simulink model "gm_sampleModel1580_4_sub"  (R2023a)
settings: Solver=VariableStepAuto  StartTime=0.0  StopTime=10.0  RelTol=1e-3
libraries: hdlsllib x3, simulink x2
settings Model: Creator=user1  LastModifiedBy=user1
settings OptimizationCC: BlockReduction=off  ConditionallyExecuteInputs=off
settings DebuggingCC: InheritedTsInSrcMsg=none

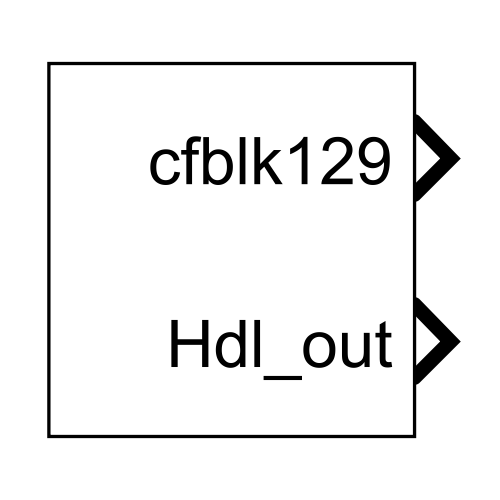
[thumbnail: Simulink's stored preview of the top-level diagram]
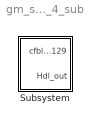
== system gm_sampleModel1580_4_sub ==
  Subsystem : Subsystem

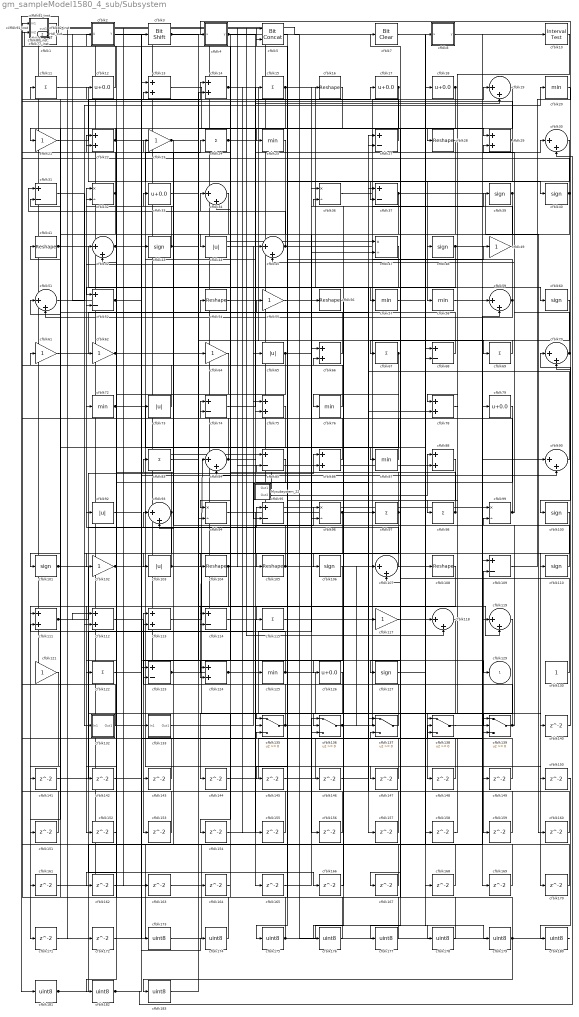
== system gm_sampleModel1580_4_sub/Subsystem ==
  Mysubsystem_22 : Subsystem
  cfblk1 : simulink/Logic and Bit Operations/Bit Clear  iBit=0
      settings: LibrarySourceBlock=|
      | hdlsllib/Logic and Bit
      | Operations/Bit Clear
  cfblk10 : hdlsllib/Logic and Bit Operations/Interval Test  IntervalClosedRight=on  uplimit=0.5  IntervalClosedLeft=on  lowlimit=-0.5  OutDataTypeStr=uint8
  cfblk{39..40,43,48,60,100..101,106,110,127} (10 alike) : Signum
  cfblk{21,23,49,55,61..62,64,102,117,121} (10 alike) : Gain  OutDataTypeStr=uint8
  cfblk{44,65,73,92,103} (5 alike) : Abs  OutDataTypeStr=uint8  SaturateOnIntegerOverflow=off
  cfblk{16,28,41,54,56,104..105,108} (8 alike) : Reshape
  cfblk{19,30,34,42,45,51,59,70,84,90,93,107,118..119} (14 alike) : Sum  Inputs=|++  OutDataTypeStr=uint8
  cfblk{27,31,37,52,68,74,85,95,109,114,123} (11 alike) : Sum  Inputs=+-  OutDataTypeStr=uint8
  cfblk{11,15,24,67,69,83,97..98,115,122} (10 alike) : Sum  Inputs=+  OutDataTypeStr=uint8
  cfblk{13..14,22,29,66,75,78,86,88,111..113,124} (13 alike) : Sum  OutDataTypeStr=uint8
  cfblk{12,17..18,33,79,126} (6 alike) : Bias  Bias=0.0  SaturateOnIntegerOverflow=off
  cfblk120_inst : Subsystem
  cfblk{20,25,57..58,72,76,87,125} (8 alike) : MinMax  OutDataTypeStr=uint8
  cfblk130 : Constant  OutDataTypeStr=uint8  SampleTime=-1
  cfblk132 : Subsystem
  cfblk133 : Subsystem
  cfblk{135..139} (5 alike) : Switch  OutDataTypeStr=uint8  SaturateOnIntegerOverflow=off  InputSameDT=off
  cfblk{140..172} (33 alike) : Delay  SampleTime=1
  cfblk{173..183} (11 alike) : DataTypeConversion  OutDataTypeStr=uint8  SaturateOnIntegerOverflow=off  RndMeth=Floor
  cfblk2 : Subsystem  mask(Detect Rise Nonnegative){vinit=double(0), InputProcessing=Elements as channels (sample based), OutDataTypeStr=uint8}
      mask prompts: vinit "Simulink:masks:InitialCondition_MP"; InputProcessing "Simulink:masks:InputProcessing_MP"; OutDataTypeStr "Simulink:masks:OutputDataType_MP"
      mask help: Simulink:masks:DetectRiseNonnegative_MD
      mask init:
      | InputProcessing = 'Elements as channels (sample based)';
      | OutDataTypeStr = 'uint8';
      | vinit = double(0);
      mask TypeOptions InputProcessing: Simulink:masks:ColumnsAsChannelsFrameBased | Simulink:masks:ElementsAsChannelsSampleBased
      mask TypeOptions OutDataTypeStr: Simulink:masks:uint8 | Simulink:masks:boolean
      mask Display: fprintf('U >= 0\n&  NOT\nU/z >= 0')
  cfblk3 : hdlsllib/Logic and Bit Operations/Bit Shift  mode=Shift Left Logical  N=0
  cfblk{32,36,47,94,96,99} (6 alike) : Product  Inputs=*/  OutDataTypeStr=uint8  RndMeth=Zero  SaturateOnIntegerOverflow=on
  cfblk4 : Subsystem  mask(Compare To Zero){relop=<=, OutDataTypeStr=uint8, ZeroCross=on}
      mask prompts: relop "Simulink:masks:Operator_MP"; OutDataTypeStr "Simulink:masks:OutputDataType_MP"; ZeroCross "Simulink:masks:EnableZerocrossingDetection_MP"
      mask help: Simulink:masks:CompareToZero_MD
      mask init:
      | OutDataTypeStr = 'uint8';
      | ZeroCross = 'on';
      | blkName = 'sampleModel1580_4_sub/Subsystem/cfblk4';
      | relop = '<=';
      | setValue = 'fixdt(0, 8)';
      mask TypeOptions relop: == | ~= | < | <= | >= | >
      mask TypeOptions OutDataTypeStr: Simulink:masks:uint8 | Simulink:masks:boolean
      mask Callback ZeroCross: sl('zeroCrossEnable', gcbh);
      mask Display: disp([relop,' 0'])
  cfblk46_inst : Subsystem
  cfblk5 : hdlsllib/Logic and Bit Operations/Bit Concat  numInputs=2
  cfblk50_inst : Subsystem
  cfblk53_inst : Subsystem
  cfblk6 : Constant  Value=0  OutDataTypeStr=uint8  SampleTime=1
  cfblk63_inst : Subsystem
  cfblk7 : simulink/Logic and Bit Operations/Bit Clear  iBit=0
      settings: LibrarySourceBlock=|
      | hdlsllib/Logic and Bit
      | Operations/Bit Clear
  cfblk71_inst : Subsystem
  cfblk77_inst : Subsystem
  cfblk8 : Subsystem  mask(Compare To Constant){relop=<=, const=double(3), OutDataTypeStr=uint8, ZeroCross=on}
      mask prompts: relop "Simulink:masks:Operator_MP"; const "Simulink:masks:ConstantValue_MP"; OutDataTypeStr "Simulink:masks:OutputDataType_MP"; ZeroCross "Simulink:masks:EnableZerocrossingDetection_MP"
      mask help: Simulink:masks:CompareToConstant_MD
      mask init:
      | OutDataTypeStr = 'uint8';
      | ZeroCross = 'on';
      | blkName = 'sampleModel1580_4_sub/Subsystem/cfblk8';
      | const = double(3);
      | const_str = '3.0';
      | const_val = double(3);
      | relop = '<=';
      | setValue = 'fixdt(0, 8)';
      | str = '<= 3';
      mask TypeOptions relop: == | ~= | < | <= | >= | >
      mask TypeOptions OutDataTypeStr: Simulink:masks:uint8 | Simulink:masks:boolean
      mask Callback ZeroCross: sl('zeroCrossEnable', gcbh);
      mask Display: disp(str)
  cfblk80_inst : Subsystem
  cfblk81_inst : Subsystem
  cfblk82_inst : Subsystem
  cfblk9 : Constant  Value=0  OutDataTypeStr=uint8  SampleTime=1
  cfblk91_inst : Subsystem
  cfblk129 : Outport  OutDataTypeStr=uint8  SampleTime=1  VectorParamsAs1DForOutWhenUnconnected=off
  Hdl_out : Outport  Port=2  OutDataTypeStr=uint8  SampleTime=1
  wires:
  Mysubsystem_22/1(Out1) -> cfblk80_inst/2(in2)
  Mysubsystem_22/2(Out2) -> cfblk88/1
  cfblk1/1 -> cfblk181/1
  cfblk10/1 -> cfblk135/1
  cfblk100/1 -> cfblk170/1
  cfblk101/1 -> cfblk86/1, cfblk136/2, cfblk166/1
  cfblk102/1 -> cfblk150/1, cfblk24/1
  cfblk103/1 -> cfblk32/1, cfblk140/1
  cfblk104/1 -> cfblk75/1, cfblk152/1
  cfblk105/1 -> cfblk33/1, cfblk61/1
  cfblk106/1 -> cfblk153/1
  cfblk107/1 -> cfblk92/1
  cfblk108/1 -> cfblk171/1
  cfblk109/1 -> cfblk4/1(u)
  cfblk11/1 -> cfblk58/1
  cfblk110/1 -> cfblk83/1
  cfblk111/1 -> cfblk95/1, cfblk112/1
  cfblk112/1 -> cfblk143/1
  cfblk113/1 -> cfblk115/1
  cfblk114/1 -> cfblk165/1
  cfblk115/1 -> cfblk49/1
  cfblk117/1 -> cfblk18/1
  cfblk118/1 -> cfblk148/1
  cfblk119/1 -> cfblk144/1
  cfblk12/1 -> cfblk82_inst/1(in1)
  cfblk120_inst/1(out1) -> cfblk91_inst/1(in1), cfblk118/2, cfblk133/1(In1)
  cfblk121/1 -> cfblk161/1
  cfblk122/1 -> cfblk3/1
  cfblk123/1 -> cfblk84/1, cfblk136/3
  cfblk124/1 -> cfblk56/1, cfblk159/1
  cfblk125/1 -> cfblk111/2, cfblk168/1
  cfblk126/1 -> cfblk154/1
  cfblk127/1 -> cfblk8/1(u)
  cfblk13/1 -> cfblk75/2
  cfblk130/1 -> cfblk85/2
  cfblk132/1(Out1) -> cfblk50_inst/1(in1)
  cfblk133/1(Out1) -> cfblk65/1
  cfblk135/1 -> cfblk54/1, cfblk147/1
  cfblk136/1 -> cfblk19/1, cfblk107/1
  cfblk137/1 -> cfblk113/1
  cfblk138/1 -> cfblk109/2
  cfblk139/1 -> cfblk123/2, cfblk99/2
  cfblk14/1 -> cfblk156/1, cfblk155/1
  cfblk140/1 -> cfblk70/1
  cfblk141/1 -> cfblk45/1
  cfblk142/1 -> cfblk90/2
  cfblk143/1 -> cfblk51/1
  cfblk144/1 -> cfblk137/3
  cfblk145/1 -> cfblk109/1
  cfblk146/1 -> cfblk27/2
  cfblk147/1 -> cfblk93/1
  cfblk148/1 -> cfblk107/2
  cfblk149/1 -> cfblk46_inst/1(in1)
  cfblk15/1 -> cfblk52/1, cfblk157/1
  cfblk150/1 -> cfblk180/1
  cfblk151/1 -> cfblk53_inst/2(in2)
  cfblk152/1 -> cfblk32/2
  cfblk153/1 -> cfblk77_inst/1(in1)
  cfblk154/1 -> cfblk96/1
  cfblk155/1 -> cfblk74/1
  cfblk156/1 -> cfblk120_inst/1(in1)
  cfblk157/1 -> cfblk137/1
  cfblk158/1 -> cfblk138/2
  cfblk159/1 -> cfblk138/3
  cfblk16/1 -> cfblk25/1
  cfblk160/1 -> cfblk36/2
  cfblk161/1 -> cfblk123/1
  cfblk162/1 -> cfblk68/1
  cfblk163/1 -> cfblk59/2
  cfblk164/1 -> cfblk84/2
  cfblk165/1 -> cfblk136/1
  cfblk166/1 -> cfblk66/2
  cfblk167/1 -> cfblk50_inst/2(in2)
  cfblk168/1 -> cfblk81_inst/2(in2)
  cfblk169/1 -> cfblk31/2
  cfblk17/1 -> cfblk34/2, cfblk101/1
  cfblk170/1 -> cfblk113/2
  cfblk171/1 -> cfblk139/2
  cfblk172/1 -> cfblk139/1
  cfblk173/1 -> cfblk79/1
  cfblk174/1 -> cfblk2/1(U)
  cfblk175/1 -> cfblk34/1, cfblk178/1, cfblk120_inst/2(in2)
  cfblk176/1 -> cfblk5/1
  cfblk177/1 -> cfblk5/2
  cfblk178/1 -> cfblk7/1
  cfblk179/1 -> cfblk41/1, cfblk183/1
  cfblk18/1 -> cfblk37/2, cfblk124/2
  cfblk180/1 -> cfblk1/1
  cfblk181/1 -> cfblk43/1, cfblk139/3
  cfblk182/1 -> cfblk30/2, cfblk174/1, cfblk135/3
  cfblk183/1 -> cfblk64/1
  cfblk19/1 -> cfblk94/1
  cfblk2/1(Y) -> cfblk173/1
  cfblk20/1 -> cfblk70/2
  cfblk21/1 -> cfblk13/2
  cfblk22/1 -> cfblk21/1, cfblk169/1
  cfblk23/1 -> cfblk93/2, cfblk28/1, cfblk119/2
  cfblk24/1 -> cfblk104/1, cfblk96/2
  cfblk25/1 -> cfblk44/1
  cfblk27/1 -> cfblk53_inst/1(in1)
  cfblk28/1 -> cfblk111/1
  cfblk29/1 -> cfblk46_inst/2(in2), cfblk145/1
  cfblk3/1 -> cfblk105/1, cfblk69/1
  cfblk30/1 -> cfblk127/1
  cfblk31/1 -> cfblk132/1(In1)
  cfblk32/1 -> cfblk77_inst/2(in2), cfblk141/1
  cfblk33/1 -> cfblk87/1
  cfblk34/1 -> cfblk94/2
  cfblk36/1 -> cfblk40/1
  cfblk37/1 -> cfblk86/2, cfblk42/2, cfblk160/1
  cfblk39/1 -> cfblk68/2, cfblk177/1
  cfblk4/1(y) -> cfblk29/1, cfblk19/2, cfblk114/2
  cfblk40/1 -> cfblk63_inst/2(in2), cfblk48/1
  cfblk41/1 -> cfblk118/1, cfblk149/1
  cfblk42/1 -> cfblk14/1, cfblk126/1
  cfblk43/1 -> cfblk22/1, cfblk129/1
  cfblk44/1 -> cfblk30/1
  cfblk45/1 -> cfblk39/1, cfblk31/1
  cfblk46_inst/1(out1) -> cfblk117/1
  cfblk47/1 -> cfblk142/1
  cfblk48/1 -> cfblk59/1, cfblk135/2
  cfblk49/1 -> cfblk36/1
  cfblk5/1 -> cfblk175/1
  cfblk50_inst/1(out1) -> cfblk97/1
  cfblk51/1 -> cfblk20/1
  cfblk52/1 -> cfblk13/1, Hdl_out/1
  cfblk53_inst/1(out1) -> cfblk88/2
  cfblk54/1 -> cfblk146/1
  cfblk55/1 -> cfblk57/1
  cfblk56/1 -> cfblk176/1
  cfblk57/1 -> cfblk60/1
  cfblk58/1 -> cfblk90/1
  cfblk59/1 -> cfblk82_inst/2(in2), cfblk51/2
  cfblk6/1 -> cfblk172/1, cfblk10/1
  cfblk60/1 -> cfblk78/1
  cfblk61/1 -> cfblk37/1
  cfblk62/1 -> cfblk14/2, cfblk12/1
  cfblk63_inst/1(out1) -> cfblk71_inst/2(in2), cfblk121/1
  cfblk64/1 -> cfblk182/1
  cfblk65/1 -> cfblk16/1, cfblk102/1
  cfblk66/1 -> cfblk23/1
  cfblk67/1 -> cfblk124/1, cfblk76/1
  cfblk68/1 -> cfblk11/1
  cfblk69/1 -> cfblk67/1
  cfblk7/1 -> cfblk179/1
  cfblk70/1 -> cfblk45/2, cfblk100/1
  cfblk71_inst/1(out1) -> cfblk85/1, cfblk164/1, cfblk163/1
  cfblk72/1 -> cfblk158/1, cfblk15/1
  cfblk73/1 -> cfblk62/1
  cfblk74/1 -> cfblk17/1
  cfblk75/1 -> cfblk151/1
  cfblk76/1 -> cfblk91_inst/2(in2)
  cfblk77_inst/1(out1) -> cfblk73/1
  cfblk78/1 -> cfblk98/1
  cfblk79/1 -> cfblk95/2
  cfblk8/1(y) -> cfblk119/1
  cfblk80_inst/1(out1) -> cfblk108/1
  cfblk81_inst/1(out1) -> cfblk125/1
  cfblk82_inst/1(out1) -> cfblk99/1
  cfblk83/1 -> cfblk55/1
  cfblk84/1 -> cfblk80_inst/1(in1), cfblk71_inst/1(in1), cfblk137/2
  cfblk85/1 -> cfblk162/1
  cfblk86/1 -> cfblk63_inst/1(in1)
  cfblk87/1 -> cfblk74/2
  cfblk88/1 -> cfblk103/1
  cfblk9/1 -> cfblk81_inst/1(in1)
  cfblk90/1 -> cfblk27/1
  cfblk91_inst/1(out1) -> cfblk47/1
  cfblk92/1 -> cfblk138/1
  cfblk93/1 -> cfblk52/2, cfblk122/1
  cfblk94/1 -> cfblk110/1
  cfblk95/1 -> cfblk47/2
  cfblk96/1 -> cfblk78/2, cfblk112/2, cfblk106/1
  cfblk97/1 -> cfblk22/2, cfblk114/1, cfblk167/1
  cfblk98/1 -> cfblk42/1, cfblk72/1
  cfblk99/1 -> cfblk66/1, cfblk29/2

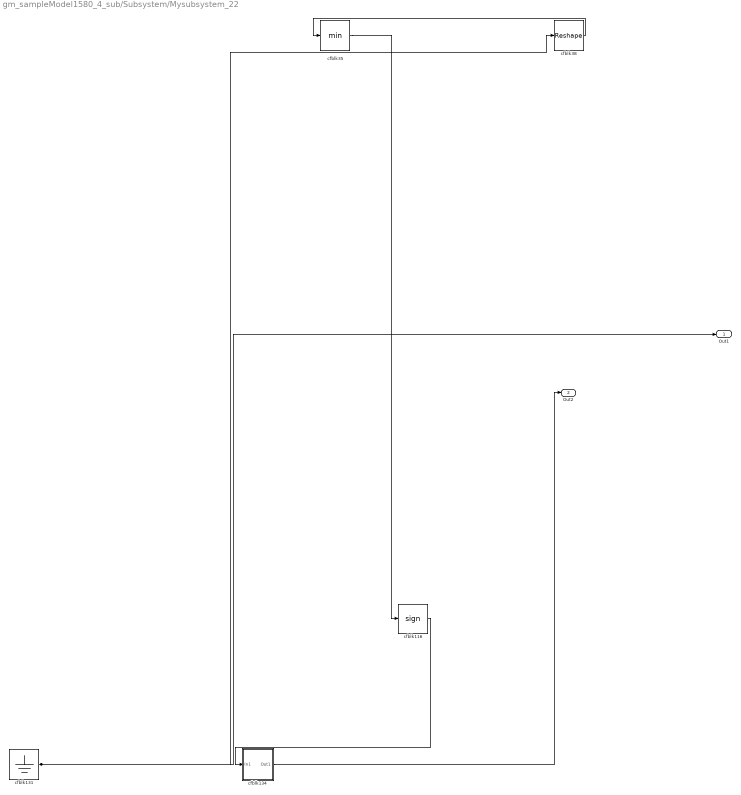
== system gm_sampleModel1580_4_sub/Subsystem/Mysubsystem_22 ==
  cfblk116 : Signum
  cfblk131 : Ground
  cfblk134 : Subsystem
  cfblk35 : MinMax
  cfblk38 : Reshape
  Out1 : Outport  SampleTime=1
  Out2 : Outport  Port=2  SampleTime=1
  wires:
  cfblk116/1 -> cfblk134/1(In1)
  cfblk131/1 -> cfblk38/1, Out1/1
  cfblk134/1(Out1) -> Out2/1
  cfblk35/1 -> cfblk116/1
  cfblk38/1 -> cfblk35/1

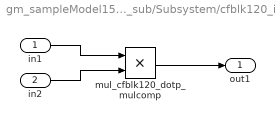
== system gm_sampleModel1580_4_sub/Subsystem/cfblk120_inst ==
  in1 : Inport  OutDataTypeStr=uint8  SampleTime=1
  in2 : Inport  Port=2  OutDataTypeStr=uint8  SampleTime=1
  mul_cfblk120_dotp_mulcomp : Product  Inputs=**  OutDataTypeStr=uint8  SampleTime=1
  out1 : Outport  OutDataTypeStr=uint8  SampleTime=1
  wires:
  in1/1 -> mul_cfblk120_dotp_mulcomp/1
  in2/1 -> mul_cfblk120_dotp_mulcomp/2
  mul_cfblk120_dotp_mulcomp/1 -> out1/1

== system gm_sampleModel1580_4_sub/Subsystem/cfblk132 ==
  In1 : Inport  OutDataTypeStr=uint8  PortDimensions=1  SampleTime=1
  Out1 : Outport  SampleTime=1
  wires:
  In1/1 -> Out1/1

== system gm_sampleModel1580_4_sub/Subsystem/cfblk133 ==
  In1 : Inport  OutDataTypeStr=uint8  PortDimensions=1  SampleTime=1
  Out1 : Outport  SampleTime=1
  wires:
  In1/1 -> Out1/1

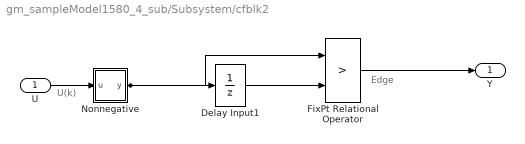
== system gm_sampleModel1580_4_sub/Subsystem/cfblk2 ==
  note: U(k)
  note: Edge
  U : Inport  OutDataTypeStr=uint8  SampleTime=1
  Delay Input1 : UnitDelay  Description=Store in Global RAM  DisableCoverage=on  InitialCondition=vinit  SampleTime=-1  HasFrameUpgradeWarning=on
  FixPt Relational Operator : RelationalOperator  Operator=>  OutDataTypeStr=fixdt(0, 8)  ZeroCross=off  InputSameDT=off
  Nonnegative : Subsystem  mask(Compare To Zero){relop=>=, OutDataTypeStr=boolean, ZeroCross=off}
      mask prompts: relop "Simulink:masks:Operator_MP"; OutDataTypeStr "Simulink:masks:OutputDataType_MP"; ZeroCross "Simulink:masks:EnableZerocrossingDetection_MP"
      mask help: Simulink:masks:CompareToZero_MD
      mask init:
      | OutDataTypeStr = 'boolean';
      | ZeroCross = 'off';
      | blkName = 'sampleModel1580_4_sub/Subsystem/cfblk2/Nonnegative';
      | relop = '>=';
      | setValue = 'boolean';
      mask TypeOptions relop: == | ~= | < | <= | >= | >
      mask TypeOptions OutDataTypeStr: Simulink:masks:uint8 | Simulink:masks:boolean
      mask Callback ZeroCross: sl('zeroCrossEnable', gcbh);
      mask Display: disp([relop,' 0'])
  Y : Outport  SampleTime=1
  wires:
  U/1 -> Nonnegative/1(u)
  Delay Input1/1 -> FixPt Relational Operator/2
  FixPt Relational Operator/1 -> Y/1
  Nonnegative/1(y) -> FixPt Relational Operator/1, Delay Input1/1

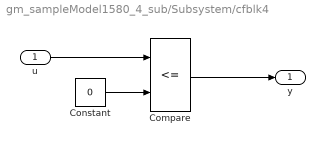
== system gm_sampleModel1580_4_sub/Subsystem/cfblk4 ==
  u : Inport  OutDataTypeStr=uint8  SampleTime=1
  Compare : RelationalOperator  Operator=<=  OutDataTypeStr=fixdt(0, 8)
  Constant : Constant  DisableCoverage=on  Value=0  OutDataTypeStr=Inherit: Inherit via back propagation  SampleTime=-1  PreserveConstantTs=on
  y : Outport  SampleTime=1
  wires:
  u/1 -> Compare/1
  Compare/1 -> y/1
  Constant/1 -> Compare/2

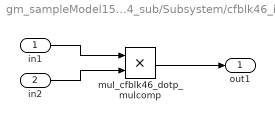
== system gm_sampleModel1580_4_sub/Subsystem/cfblk46_inst ==
  in1 : Inport  OutDataTypeStr=uint8  SampleTime=1
  in2 : Inport  Port=2  OutDataTypeStr=uint8  SampleTime=1
  mul_cfblk46_dotp_mulcomp : Product  Inputs=**  OutDataTypeStr=uint8  SampleTime=1
  out1 : Outport  OutDataTypeStr=uint8  SampleTime=1
  wires:
  in1/1 -> mul_cfblk46_dotp_mulcomp/1
  in2/1 -> mul_cfblk46_dotp_mulcomp/2
  mul_cfblk46_dotp_mulcomp/1 -> out1/1

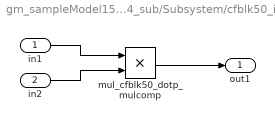
== system gm_sampleModel1580_4_sub/Subsystem/cfblk50_inst ==
  in1 : Inport  OutDataTypeStr=uint8  SampleTime=1
  in2 : Inport  Port=2  OutDataTypeStr=uint8  SampleTime=1
  mul_cfblk50_dotp_mulcomp : Product  Inputs=**  OutDataTypeStr=uint8  SampleTime=1
  out1 : Outport  OutDataTypeStr=uint8  SampleTime=1
  wires:
  in1/1 -> mul_cfblk50_dotp_mulcomp/1
  in2/1 -> mul_cfblk50_dotp_mulcomp/2
  mul_cfblk50_dotp_mulcomp/1 -> out1/1

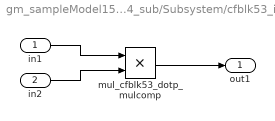
== system gm_sampleModel1580_4_sub/Subsystem/cfblk53_inst ==
  in1 : Inport  OutDataTypeStr=uint8  SampleTime=1
  in2 : Inport  Port=2  OutDataTypeStr=uint8  SampleTime=1
  mul_cfblk53_dotp_mulcomp : Product  Inputs=**  OutDataTypeStr=uint8  SampleTime=1
  out1 : Outport  OutDataTypeStr=uint8  SampleTime=1
  wires:
  in1/1 -> mul_cfblk53_dotp_mulcomp/1
  in2/1 -> mul_cfblk53_dotp_mulcomp/2
  mul_cfblk53_dotp_mulcomp/1 -> out1/1

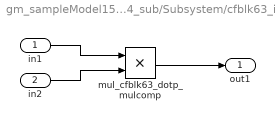
== system gm_sampleModel1580_4_sub/Subsystem/cfblk63_inst ==
  in1 : Inport  OutDataTypeStr=uint8  SampleTime=1
  in2 : Inport  Port=2  OutDataTypeStr=uint8  SampleTime=1
  mul_cfblk63_dotp_mulcomp : Product  Inputs=**  OutDataTypeStr=uint8  SampleTime=1
  out1 : Outport  OutDataTypeStr=uint8  SampleTime=1
  wires:
  in1/1 -> mul_cfblk63_dotp_mulcomp/1
  in2/1 -> mul_cfblk63_dotp_mulcomp/2
  mul_cfblk63_dotp_mulcomp/1 -> out1/1

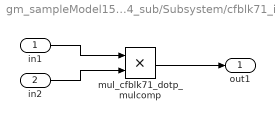
== system gm_sampleModel1580_4_sub/Subsystem/cfblk71_inst ==
  in1 : Inport  OutDataTypeStr=uint8  SampleTime=1
  in2 : Inport  Port=2  OutDataTypeStr=uint8  SampleTime=1
  mul_cfblk71_dotp_mulcomp : Product  Inputs=**  OutDataTypeStr=uint8  SampleTime=1
  out1 : Outport  OutDataTypeStr=uint8  SampleTime=1
  wires:
  in1/1 -> mul_cfblk71_dotp_mulcomp/1
  in2/1 -> mul_cfblk71_dotp_mulcomp/2
  mul_cfblk71_dotp_mulcomp/1 -> out1/1

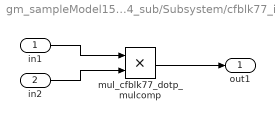
== system gm_sampleModel1580_4_sub/Subsystem/cfblk77_inst ==
  in1 : Inport  OutDataTypeStr=uint8  SampleTime=1
  in2 : Inport  Port=2  OutDataTypeStr=uint8  SampleTime=1
  mul_cfblk77_dotp_mulcomp : Product  Inputs=**  OutDataTypeStr=uint8  SampleTime=1
  out1 : Outport  OutDataTypeStr=uint8  SampleTime=1
  wires:
  in1/1 -> mul_cfblk77_dotp_mulcomp/1
  in2/1 -> mul_cfblk77_dotp_mulcomp/2
  mul_cfblk77_dotp_mulcomp/1 -> out1/1

== system gm_sampleModel1580_4_sub/Subsystem/cfblk8 ==
  u : Inport  OutDataTypeStr=uint8  SampleTime=1
  Compare : RelationalOperator  Operator=<=  OutDataTypeStr=fixdt(0, 8)
  Constant : Constant  DisableCoverage=on  Value=const  OutDataTypeStr=Inherit: Inherit via back propagation  SampleTime=-1
  y : Outport  SampleTime=1
  wires:
  u/1 -> Compare/1
  Compare/1 -> y/1
  Constant/1 -> Compare/2

== system gm_sampleModel1580_4_sub/Subsystem/cfblk80_inst ==
  in1 : Inport  OutDataTypeStr=uint8  SampleTime=1
  in2 : Inport  Port=2  OutDataTypeStr=uint8  SampleTime=1
  mul_cfblk80_dotp_mulcomp : Product  Inputs=**  OutDataTypeStr=uint8  SampleTime=1
  out1 : Outport  OutDataTypeStr=uint8  SampleTime=1
  wires:
  in1/1 -> mul_cfblk80_dotp_mulcomp/1
  in2/1 -> mul_cfblk80_dotp_mulcomp/2
  mul_cfblk80_dotp_mulcomp/1 -> out1/1

== system gm_sampleModel1580_4_sub/Subsystem/cfblk81_inst ==
  in1 : Inport  OutDataTypeStr=uint8  SampleTime=1
  in2 : Inport  Port=2  OutDataTypeStr=uint8  SampleTime=1
  mul_cfblk81_dotp_mulcomp : Product  Inputs=**  OutDataTypeStr=uint8  SampleTime=1
  out1 : Outport  OutDataTypeStr=uint8  SampleTime=1
  wires:
  in1/1 -> mul_cfblk81_dotp_mulcomp/1
  in2/1 -> mul_cfblk81_dotp_mulcomp/2
  mul_cfblk81_dotp_mulcomp/1 -> out1/1

== system gm_sampleModel1580_4_sub/Subsystem/cfblk82_inst ==
  in1 : Inport  OutDataTypeStr=uint8  SampleTime=1
  in2 : Inport  Port=2  OutDataTypeStr=uint8  SampleTime=1
  mul_cfblk82_dotp_mulcomp : Product  Inputs=**  OutDataTypeStr=uint8  SampleTime=1
  out1 : Outport  OutDataTypeStr=uint8  SampleTime=1
  wires:
  in1/1 -> mul_cfblk82_dotp_mulcomp/1
  in2/1 -> mul_cfblk82_dotp_mulcomp/2
  mul_cfblk82_dotp_mulcomp/1 -> out1/1

== system gm_sampleModel1580_4_sub/Subsystem/cfblk91_inst ==
  in1 : Inport  OutDataTypeStr=uint8  SampleTime=1
  in2 : Inport  Port=2  OutDataTypeStr=uint8  SampleTime=1
  mul_cfblk91_dotp_mulcomp : Product  Inputs=**  OutDataTypeStr=uint8  SampleTime=1
  out1 : Outport  OutDataTypeStr=uint8  SampleTime=1
  wires:
  in1/1 -> mul_cfblk91_dotp_mulcomp/1
  in2/1 -> mul_cfblk91_dotp_mulcomp/2
  mul_cfblk91_dotp_mulcomp/1 -> out1/1

== system gm_sampleModel1580_4_sub/Subsystem/Mysubsystem_22/cfblk134 ==
  In1 : Inport  OutDataTypeStr=uint8  PortDimensions=1  SampleTime=1
  Out1 : Outport  SampleTime=1
  wires:
  In1/1 -> Out1/1

== system gm_sampleModel1580_4_sub/Subsystem/cfblk2/Nonnegative ==
  u : Inport  OutDataTypeStr=uint8  SampleTime=1
  Compare : RelationalOperator  OutDataTypeStr=boolean  ZeroCross=off
  Constant : Constant  DisableCoverage=on  Value=0  OutDataTypeStr=Inherit: Inherit via back propagation  SampleTime=-1  PreserveConstantTs=on
  y : Outport  SampleTime=1
  wires:
  u/1 -> Compare/1
  Compare/1 -> y/1
  Constant/1 -> Compare/2
